simulink model "irep_single_axis"  (Simulink 7.5)
settings: Solver=ode3  StartTime=0.0  StopTime=inf  FixedStep=dt  RelTol=1e-3
InitFcn:
  | IREPOLD_DEPENDENCY
  | init_omni
  | init_filters
  | init_invivo
  | init_telemanipulation
  | init_parker_xyz
  | init_magnetic_tracker
  | init_loadcell
  | init_scopes
  | init_homing
  | init_force_control
  | ATI_Init_nano17
undefined symbols (not defined in the file): A, ATI_torque_convert_to_Nmm, counter_offset, DiscIntNeverNeededParam, dt, encoder_counts, filter_coeffs_ATI, filter_coeffs_ATI_bias, gear_ratio, HomingFineEps, HomingRoughEps, HomingRoughVelocity, inv_T, joystick_filter_coeffs, K_d, K_i, K_p, left_arm_home_voltage, N_ATI, N_ATI_bias, N_joystick, N_pots, pots_filter_coeffs, quadrature_mode, right_arm_home_voltage, RightArmHomingDirectionVector, RightArmHomingIntGain, screw_pitch
libraries: xpcconteclib x23, xpcmeasurementcomputinglib x17, xpclib x11, simulink x8, dspswit3 x4, dspsigops x1, powerlib_extras x1
(part 3 of 3)

== matlab function Trajectory Planner/Left Arm/Low Level/Home Procedure/Fine_Rough_Homing_Switch ==
  data: EnableFineHoming output double; error input double; dt input double; q_des output double; ERROR_eps input double; HomingVel input double; q_cur input double; HomedJoint output boolean; PrevHomedJoint input boolean
function [EnableFineHoming,q_des,HomedJoint] = fcn(error, dt,ERROR_eps,HomingVel,q_cur,PrevHomedJoint)
%#eml
%   By Long Wang, 2015/1/20
%   Input:
%       error       -> the current error in potentiometers
%       ERROR_eps   -> the tolenrace defined in potentiometers which will determine if within rough control range 
%       q_cur       -> the previous command
%       PrevHomedJoint  -> if homed detected from the previous time step
%       HomingVel       -> the joint velocity to command if the joint is rough homing mode
HomedJoint = (abs(error)<ERROR_eps);
HomedJoint = (HomedJoint|PrevHomedJoint); 
%   if the joint was detected homed previously, it will be forever seen as homed
%   to avoid noise on pots.
if sum(HomedJoint)==9
    % all joints are in rough homing control range, need to use fine homing
    q_des = q_cur; % stays the previous command
    EnableFineHoming = 1;
else
    %   not all joints are in rough homing control range
    %   the ones which are not, need to give constant velocity command
    %   And the other joints will be waiting untill all the joints are in Fine Homing mode
    EnableFineHoming = 0;
    velocity = (1-HomedJoint).*sign(error).*HomingVel; 
    q_des = q_cur + velocity*dt;
end

== matlab function Trajectory Planner/Left Arm/Low Level/Home Procedure/Homing Completion ==
  data: u input double; Homed output double; EPS input double
function Homed = fcn(u,EPS)
%#eml
u = abs(u);
Homed = (u<=EPS);

== matlab function Trajectory Planner/Left Arm/Low Level/Home Procedure2/Homing Completion ==
  data: u input double; y output double
function y = fcn(u)
%#eml
y = zeros(9,1);
u = abs(u);
if u(1) <= 0.002
    y(1) = 1;
end
if u(2) <= 0.002
    y(2) = 1;
end
if u(3) <= 0.002
    y(3) = 1;
end
if u(4) <= 0.002
    y(4) = 1;
end
if u(5) <= 0.002
    y(5) = 1;
end
if u(6) <= 0.002
    y(6) = 1;
end
if u(7) <= 0.002
    y(7) = 1;
end
if u(8) <= 0.002
    y(8) = 1;
end
if u(9) <= 0.002
    y(9) = 1;
end
